simulink model "RL_FA_controller_5ESD0"  (R2024b)
settings: Solver=VariableStepAuto  StartTime=0.0  StopTime=10.0  RelTol=1e-3
values from neighbouring files (symbols this model uses):
  reset = 0    [RL_FA_controller_5ESD0.mat]    (also in TunableParams.m)
  resetEnc = 0    [RL_FA_controller_5ESD0.mat]    (also in TunableParams.m)
  SigGen_Amplitude = 0    [RL_FA_controller_5ESD0.mat]    (also in TunableParams.m)
  SigGen_Frequency = 1    [RL_FA_controller_5ESD0.mat]    (also in TunableParams.m)
libraries: cstblocks x2, simulink x2
settings Model: Creator=whendrix  LastModifiedBy=danieltyukov
settings SolverCC: AlgebraicLoopSolver=TrustRegion
settings DebuggingCC: UnconnectedInputMsg=warning  UnconnectedOutputMsg=warning  UnconnectedLineMsg=warning
settings ModelReferenceCC: EnableRefExpFcnMdlSchedulingChecks=on
settings RTWCC: GPUComputeCapability=3.5  DLArmComputeVersion=19.05

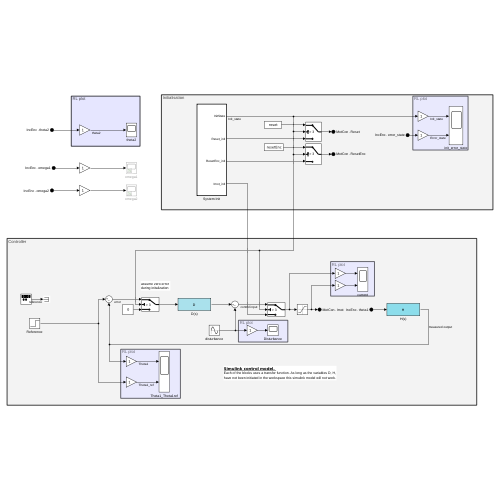
[thumbnail: Simulink's stored preview of the top-level diagram]
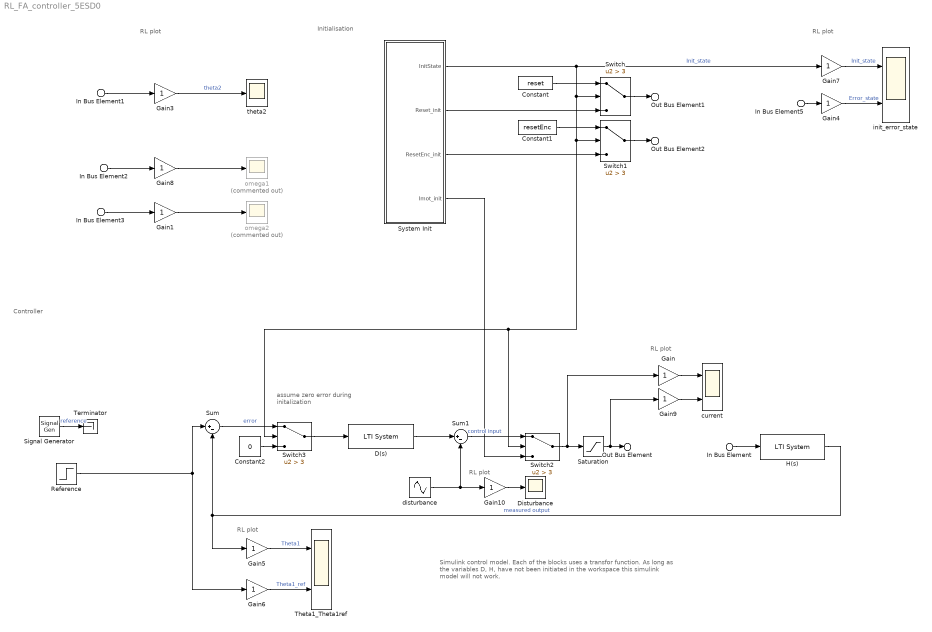
== system RL_FA_controller_5ESD0 ==
  note: RL plot
  note: RL plot
  note: RL plot
  note: RL plot
  note: RL plot
  note: assume zero error
      | during initalization
  note: Simulink control model.
      | Each of the blocks uses a transfor function. As long as the variables D, H,
      | have not been initiated in the workspace this simulink model will not work.
  note: Controller
  note: Initialisation
  In Bus Element5 : Inport  PortName=IncEnc  Element=error_state
  In Bus Element : Inport  PortName=IncEnc  Element=theta1
  In Bus Element2 : Inport  PortName=IncEnc  Element=omega1
  In Bus Element1 : Inport  PortName=IncEnc  Element=theta2
  In Bus Element3 : Inport  PortName=IncEnc  Element=omega2
  Constant : Constant  Value=reset
  Constant1 : Constant  Value=resetEnc
  Constant2 : Constant  Value=0
  D(s) : cstblocks/LTI System  sys=D  IC=[]  PadeOrder=0
  Disturbance : Scope
  Gain{,1,3..10} (10 alike) : Gain
  H(s) : cstblocks/LTI System  sys=H  IC=[]  PadeOrder=0
  Reference : Step  Time=7  After=40
  Saturation : Saturate  UpperLimit=1.83  LowerLimit=-1.83
  Signal Generator : SignalGenerator  WaveForm=square  Amplitude=SigGen_Amplitude  Frequency=SigGen_Frequency
  Sum : Sum  Inputs=|+-
  Sum1 : Sum  Inputs=|+-
  Switch{,1..3} (4 alike) : Switch  Criteria=u2 > Threshold  Threshold=3  SaturateOnIntegerOverflow=off  InputSameDT=off
  System Init : Subsystem  TreatAsAtomicUnit=on
  Terminator : Terminator
  Theta1_Theta1ref : Scope  NumInputPorts=2
  current : Scope  NumInputPorts=2
  disturbance : Sin  Amplitude=0  Frequency=20
  init_error_state : Scope  NumInputPorts=2
  omega1 : Scope  Commented=on
  omega2 : Scope  Commented=on
  theta2 : Scope
  Out Bus Element2 : Outport  PortName=MotCon  Element=ResetEnc
  Out Bus Element : Outport  PortName=MotCon  Element=Imot
  Out Bus Element1 : Outport  PortName=MotCon  Element=Reset
  wires:
  In Bus Element3/1 -> Gain1/1
  In Bus Element5/1 -> Gain4/1
  Switch/1 -> Out Bus Element1/1
  Switch1/1 -> Out Bus Element2/1
  Constant/1 -> Switch/1
  Constant1/1 -> Switch1/1
  System Init/2(Reset_init) -> Switch/3
  System Init/3(ResetEnc_init) -> Switch1/3
  System Init/4(Imot_init) -> Switch2/3
  disturbance/1 -> Sum1/2, Gain10/1
  Switch2/1 -> Gain/1, Saturation/1
  In Bus Element/1 -> H(s)/1
  System Init/1(InitState) -> Switch3/2, Switch2/2, Switch1/2, Switch/2, Gain7/1  "Init_state"
  Sum/1 -> Switch3/1  "error"
  H(s)/1 -> Sum/2, Gain5/1  "measured output"
  Switch3/1 -> D(s)/1
  Constant2/1 -> Switch3/3
  Reference/1 -> Sum/1, Gain6/1
  In Bus Element1/1 -> Gain3/1
  Gain/1 -> current/1
  Gain1/1 -> omega2/1
  Gain3/1 -> theta2/1  "theta2"
  Gain5/1 -> Theta1_Theta1ref/1  "Theta1"
  Gain6/1 -> Theta1_Theta1ref/2  "Theta1_ref"
  Saturation/1 -> Gain9/1, Out Bus Element/1
  Gain7/1 -> init_error_state/1  "Init_state"
  Gain4/1 -> init_error_state/2  "Error_state"
  D(s)/1 -> Sum1/1
  Gain9/1 -> current/2
  Sum1/1 -> Switch2/1  "control input"
  Gain10/1 -> Disturbance/1
  Gain8/1 -> omega1/1
  In Bus Element2/1 -> Gain8/1
  Signal Generator/1 -> Terminator/1  "reference"

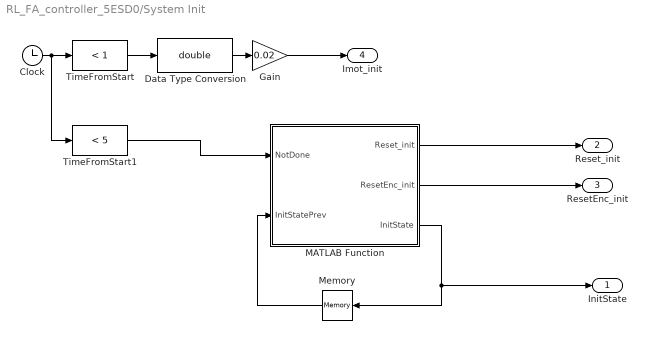
== system RL_FA_controller_5ESD0/System Init ==
  Clock : Clock
  Data Type Conversion : DataTypeConversion  OutDataTypeStr=double  SaturateOnIntegerOverflow=off  RndMeth=Floor
  Gain : Gain  Gain=0.02
  MATLAB Function : MATLAB Function  TreatAsAtomicUnit=on
  Memory : Memory
  TimeFromStart : simulink/Logic and Bit Operations/Compare To Constant  relop=<  const=1  OutDataTypeStr=boolean
  TimeFromStart1 : simulink/Logic and Bit Operations/Compare To Constant  relop=<  const=5  OutDataTypeStr=boolean
  InitState : Outport
  Reset_init : Outport  Port=2
  ResetEnc_init : Outport  Port=3
  Imot_init : Outport  Port=4
  wires:
  Clock/1 -> TimeFromStart1/1, TimeFromStart/1
  Gain/1 -> Imot_init/1
  Data Type Conversion/1 -> Gain/1
  TimeFromStart/1 -> Data Type Conversion/1
  MATLAB Function/3(InitState) -> Memory/1, InitState/1
  Memory/1 -> MATLAB Function/2(InitStatePrev)
  MATLAB Function/1(Reset_init) -> Reset_init/1
  MATLAB Function/2(ResetEnc_init) -> ResetEnc_init/1
  TimeFromStart1/1 -> MATLAB Function/1(NotDone)

== matlab function RL_FA_controller_5ESD0/System Init/MATLAB Function ==
  data: NotDone input; InitStatePrev input; Reset_init output; ResetEnc_init output; InitState output
function [Reset_init, ResetEnc_init, InitState] = fcn(NotDone,InitStatePrev)

InitState=InitStatePrev;

switch NotDone
    case 1
    InitState=0
    Reset_init=0;
    ResetEnc_init=0;
    case 0
        switch InitState
            case 0
            ResetEnc_init=1;
            Reset_init=0;
            InitState=1;
            case 1
            ResetEnc_init=0;
            Reset_init=1;
            InitState=2;
            case 2
            ResetEnc_init=0;
            Reset_init=0;
            InitState=3;
            case 3
            ResetEnc_init=0;
            Reset_init=0;
            InitState=4; 
            case 4
            ResetEnc_init=0;
            Reset_init=0;
            InitState=4;   
            otherwise
            ResetEnc_init=0;
            Reset_init=0;  
        end
    otherwise
        ResetEnc_init=0;
        Reset_init=0;
end
